simulink model "dspcelpcoder"  (Simulink 6.0)
settings: Solver=FixedStepDiscrete  SolverMode=SingleTasking  StartTime=0.0  StopTime=3  RelTol=1e-3
PreLoadFcn:
  | load lpcvocoder.mat;
values from neighbouring files (symbols this model uses):
  D = var(Noisef)    [lmsxy.m]
  Speech = [0.139446526672 0.138625044925 0.138111618832 0.138471017097 0.138316989269 0.138625044925 0.138419674488 0.137854905786 0.138419674488 0.138111618832 0.138573702316 0.138881757971 ... (24000 elements, 24000x1)]    [lpcvocoder.mat]
undefined symbols (not defined in the file or in its folder): jet, magnitude, poly2lsf
libraries: simulink x25, dspindex x17, dspcelplib x14, dsparch4 x12, dspquant2 x10, dspstat3 x10, dspsrcs4 x8, dspbuff3 x8, dspsigops x7, dspmtrx3 x6, dsplp x5, dspobslib x4
(part 3 of 3)

== system dspcelpcoder/CELP Decoder/Subframe Synthesis/Reconstruction of  Speech Subframe/Reconstruction of  Pitch Residual Signal/replace 4 selected samples by their sign and set others to zero/DocBlock ==
  EmptySubsystem : Subsystem  PropExecContextAcrossSSBoundary=on

== system dspcelpcoder/CELP Encoder/Frame Analysis/LSF Vector Quantization/LSF Split VQ./Split vector quantization of LSF/EmptySubsystem ==

== system dspcelpcoder/CELP Encoder/Frame Analysis/LSF Vector Quantization/Paliwal Weight  Computation/Calculation of Perceptual  Weighting Factors/EmptySubsystem ==

== system dspcelpcoder/CELP Encoder/Subframe Analysis/Innovation signal quantization/Searching for FCB pulse  positions and FCB gain/Optimal Features/Local maxima detector ==
  note: Note: The 'Running Maximum' block
      | exploits the reset option in 'For' iterator
  Err : Inport  LatchInput=off
  Relational Operator1 : RelationalOperator  Operator===  LogicOutDataTypeMode=Boolean  InputSameDT=on
  Running Maximum : dspstat3/Maximum  DialogController=dspDDGCreate  DialogControllerArgs=DataTag19  fcn=Running  reset=None  roundingMode=Floor  overflowMode=off
  Flag : Outport
  wires:
  Err/1 -> Running Maximum/1, Relational Operator1/1
  Running Maximum/1 -> Relational Operator1/2
  Relational Operator1/1 -> Flag/1

== system dspcelpcoder/CELP Encoder/Subframe Analysis/Innovation signal quantization/Searching for FCB pulse  positions and FCB gain/Searching for FCB features/EmptySubsystem ==

== system dspcelpcoder/CELP Encoder/Subframe Analysis/Innovation signal quantization/filter/DocBlock/EmptySubsystem ==

== system dspcelpcoder/CELP Encoder/Subframe Analysis/Pitch Estimation/Open loop  Pitch estimation/Open Loop Pitch Estimation/EmptySubsystem ==

== system dspcelpcoder/CELP Decoder/Subframe Synthesis/Reconstruction of  Speech Subframe/Reconstruction of  Pitch Residual Signal/replace 4 selected samples by their sign and set others to zero/DocBlock/EmptySubsystem ==
